simulink model "MOBATSim"  (R2020a)
settings: Solver=VariableStepAuto  StartTime=0.0  StopTime=20  FixedStep=0.01  RelTol=1e-3
undefined symbols (not defined in the file): default_spacing, FI_distance, FI_speed, max_ac, meters, min_ac, SafeDistance, Sim_Ts, simSpeed, time_gap, Ts, v_set, Vehicle1, Vehicle10, Vehicle2, Vehicle3, Vehicle4, Vehicle5, Vehicle6, Vehicle7, Vehicle8, Vehicle9, verr_gain, vx_gain, xerr_gain
libraries: simulink x32, mpcadaslib x1, robotalgslib x1
(part 3 of 4)

== system MOBATSim/Vehicle Model 9/Longitudinal Speed Control ==
  note: Here the measured speed and the actual speed are the same
      | but it is designed to include the effects of the measurement errors
  note: The vehicle calculates the speed difference between the actual speed and the reference speed, then generates the acceleration command accordingly.
  Speed Reference : Inport
  Inter Vehicular Distance : Inport  Port=2
  Lead Speed : Inport  Port=3
  Driving Mode : Inport  Port=4
  Dist2Stop : Inport  Port=5
  Acceleration Command : Subsystem
  Distance to Stop Controller : Subsystem
  Platoon Controller : Subsystem
  Reference speed according to the driving mode : Subsystem
  Signal Specification1 : SignalSpecification  Dimensions=1
  Sum13 : Sum  Inputs=|+-
  Vehicle Dynamic Model : Subsystem
  Actual Speed : Outport  VectorParamsAs1DForOutWhenUnconnected=off
  Measured Speed : Outport  Port=2  VectorParamsAs1DForOutWhenUnconnected=off
  wires:
  Platoon Controller/1(ref speed) -> Distance to Stop Controller/1(Speed Ref from Platoon), Reference speed according to the driving mode/3(In3)
  Lead Speed/1 -> Platoon Controller/2(Lead Speed)
  Driving Mode/1 -> Acceleration Command/1(Driving Mode), Reference speed according to the driving mode/1(In1)
  Signal Specification1/1 -> Actual Speed/1
  Sum13/1 -> Acceleration Command/2(Speed Error)
  Inter Vehicular Distance/1 -> Platoon Controller/1(Inter Vehicular Distance)
  Dist2Stop/1 -> Distance to Stop Controller/2(Distance to Stop)
  Speed Reference/1 -> Reference speed according to the driving mode/2(In2)
  Distance to Stop Controller/1(ref speed) -> Reference speed according to the driving mode/4(In4)
  Reference speed according to the driving mode/1(Out1) -> Sum13/1
  Vehicle Dynamic Model/1(Vehicle Speed) -> Signal Specification1/1, Acceleration Command/3(Actual Speed), Sum13/2, Platoon Controller/3(Vehicle Speed), Measured Speed/1
  Acceleration Command/1(Acceleration Command) -> Vehicle Dynamic Model/1(Acceleration Command)

== system MOBATSim/Vehicle Model 1/Longitudinal Speed Control/Acceleration Command ==
  Driving Mode : Inport
  Speed Error : Inport  Port=2
  Actual Speed : Inport  Port=3
  Emergency Brake : Constant  Value=MinDeceleration
  Gear Logic : Stateflow chart  TreatAsAtomicUnit=on
  Multiport Switch3 : MultiPortSwitch  Inputs=4
  Saturation Dynamic : simulink/Discontinuities/Saturation Dynamic  OutMin=[]  OutMax=[]  OutDataTypeStr=Inherit: Same as second input  OutDataType=fixdt(1, 16)  OutScaling=2^-10  DoSatur=off
  Acceleration Command : Outport  VectorParamsAs1DForOutWhenUnconnected=off
  wires:
  Driving Mode/1 -> Multiport Switch3/1
  Speed Error/1 -> Saturation Dynamic/2
  Emergency Brake/1 -> Saturation Dynamic/3, Multiport Switch3/4
  Saturation Dynamic/1 -> Multiport Switch3/5, Multiport Switch3/2, Multiport Switch3/3
  Actual Speed/1 -> Gear Logic/1(speed)
  Multiport Switch3/1 -> Acceleration Command/1
  Gear Logic/1(maxAcc) -> Saturation Dynamic/1

== system MOBATSim/Vehicle Model 1/Longitudinal Speed Control/Distance to Stop Controller ==
  Speed Ref from Platoon : Inport
  Distance to Stop : Inport  Port=2
  Gain : Gain  Gain=0.02
  Multiport Switch2 : MultiPortSwitch  DataPortOrder=Zero-based contiguous  Inputs=2  zeroidx=on
  Relational Operator : RelationalOperator  Operator=<=  OutDataTypeStr=boolean  RndMeth=Simplest
  ref speed : Outport  VectorParamsAs1DForOutWhenUnconnected=off
  wires:
  Distance to Stop/1 -> Gain/1
  Speed Ref from Platoon/1 -> Relational Operator/1, Multiport Switch2/3
  Gain/1 -> Relational Operator/2, Multiport Switch2/2
  Multiport Switch2/1 -> ref speed/1
  Relational Operator/1 -> Multiport Switch2/1

== system MOBATSim/Vehicle Model 1/Longitudinal Speed Control/Platoon Controller ==
  Inter Vehicular Distance : Inport
  Lead Speed : Inport  Port=2
  Vehicle Speed : Inport  Port=3
  Compare To Constant : simulink/Logic and Bit Operations/Compare To Constant  relop=>  const=2  OutDataTypeStr=uint8
  Constant : Constant  Value=meters
  Gain : Gain  Gain=1.4
  Multiport Switch : MultiPortSwitch  DataPortOrder=Zero-based contiguous  Inputs=2  zeroidx=on
  PID Controller5 : simulink/Continuous/PID Controller  Controller=PID  Form=Parallel  TimeDomain=Continuous-time  UseExternalTs=off  SampleTime=-1  IntegratorMethod=Forward Euler  FilterMethod=Forward Euler  ControllerParametersSource=internal  P=2.0341199375219  I=0.0356576460366845  D=2.08363010404189  UseFilter=on  N=233.214579742572  TunerSelectOption=Transfer Function Based (PID Tuner App)  InitialConditionSource=internal  InitialConditionForIntegrator=0  InitialConditionForFilter=0  DifferentiatorICPrevScaledInput=0  ExternalReset=none  TrackingMode=off  Kt=1  LimitOutput=on  UpperSaturationLimit=100  LowerSaturationLimit=-100  LinearizeAsGain=on  AntiWindupMode=clamping  Kb=1  POutMin=[]  POutMax=[]  IOutMin=[]  IOutMax=[]  DOutMin=[]  DOutMax=[]  NOutMin=[]  NOutMax=[]  SumOutMin=[]  SumOutMax=[]  SaturationOutMin=[]  SaturationOutMax=[]  PParamMin=[]  PParamMax=[]  IParamMin=[]  IParamMax=[]  DParamMin=[]  DParamMax=[]  NParamMin=[]  NParamMax=[]  KbParamMin=[]  KbParamMax=[]  KtParamMin=[]  KtParamMax=[]  KbOutMin=[]  KbOutMax=[]  KtOutMin=[]  KtOutMax=[]  IntegratorOutMin=[]  IntegratorOutMax=[]  FilterOutMin=[]  FilterOutMax=[]  SumI1OutMin=[]  SumI1OutMax=[]  SumI2OutMin=[]  SumI2OutMax=[]  SumI3OutMin=[]  SumI3OutMax=[]  SumI4OutMin=[]  SumI4OutMax=[]  SumDOutMin=[]  SumDOutMax=[]  DifferentiatorOutMin=[]  DifferentiatorOutMax=[]  FilterDiffOutCoefMin=[]  FilterDiffOutCoefMax=[]  ReciprocalOutMin=[]  ReciprocalOutMax=[]  SumDenOutMin=[]  SumDenOutMax=[]  SumNumOutMin=[]  SumNumOutMax=[]  DivideOutMin=[]  DivideOutMax=[]  UdiffTsProdOutMin=[]  UdiffTsProdOutMax=[]  NTsProdOutMin=[]  NTsProdOutMax=[]  UintegralTsProdOutMin=[]  UintegralTsProdOutMax=[]  UngainTsProdOutMin=[]  UngainTsProdOutMax=[]  IntegratorContinuousStateAttributes=''  IntegratorStateMustResolveToSignalObject=off  IntegratorRTWStateStorageClass=Auto  FilterContinuousStateAttributes=''  FilterStateMustResolveToSignalObject=off  FilterRTWStateStorageClass=Auto  ParallelPVariant=InternalParameters  IdealPVariant=Disabled  IVariant=InternalParameters  DVariant=InternalParameters  IntegratorVariant=Continuous  SatVariant=Enabled  AWVariant=ContClampingParallel  PCopyVariant=Disabled  TRVariant=Disabled  FdbkBlocksVariant=Forward  IdealPFdbkVariant=Disabled  SatFdbkVariant=Disabled  DerivativeFilterVariant=ContFilter  NVariant=InternalParameters  NCopyVariant=Disabled  FilterICVariant=InternalICsFilter  IntegratorICVariant=InternalICs  ExternalResetVariant=Disabled  TRSumVariant=Passthrough  SumFdbkVariant=Disabled  SumVariant=Sum_PID  TsampFilterVariant=InternalTs  TsampNgainVariant=Passthrough  TsampIntegralVariant=Passthrough
  Sum : Sum  Inputs=|-+
  Sum1 : Sum  Inputs=|++
  Sum2 : Sum  Inputs=|+-
  Transfer Fcn : TransferFcn  Numerator=[0.05]  Denominator=[1 2]
  ref speed : Outport  VectorParamsAs1DForOutWhenUnconnected=off
  wires:
  Transfer Fcn/1 -> PID Controller5/1
  Vehicle Speed/1 -> Gain/1, Sum/1
  PID Controller5/1 -> Multiport Switch/2
  Sum/1 -> Compare To Constant/1
  Multiport Switch/1 -> ref speed/1
  Compare To Constant/1 -> Multiport Switch/1
  Lead Speed/1 -> Sum/2, Multiport Switch/3
  Constant/1 -> Sum1/1
  Sum1/1 -> Sum2/2
  Gain/1 -> Sum1/2
  Sum2/1 -> Transfer Fcn/1
  Inter Vehicular Distance/1 -> Sum2/1

== system MOBATSim/Vehicle Model 1/Longitudinal Speed Control/Reference speed according to the driving mode ==
  In1 : Inport
  In2 : Inport  Port=2
  In3 : Inport  Port=3
  In4 : Inport  Port=4
  Constant1 : Constant  Value=0
  Max Speed : Saturate  UpperLimit=maxSpeed  LowerLimit=-100
  Multiport Switch : MultiPortSwitch  Inputs=4
  Out1 : Outport
  wires:
  Constant1/1 -> Multiport Switch/4
  Multiport Switch/1 -> Max Speed/1
  In1/1 -> Multiport Switch/1
  In3/1 -> Multiport Switch/3
  In2/1 -> Multiport Switch/2
  Max Speed/1 -> Out1/1
  In4/1 -> Multiport Switch/5

== system MOBATSim/Vehicle Model 1/Longitudinal Speed Control/Vehicle Dynamic Model ==
  Acceleration Command : Inport
  Integrator : Integrator  LimitOutput=on  LowerSaturationLimit=0
  Vehicle Acc to Speed Dynamics : TransferFcn  Denominator=[0.5 1]
  Vehicle Speed : Outport
  wires:
  Vehicle Acc to Speed Dynamics/1 -> Integrator/1
  Integrator/1 -> Vehicle Speed/1
  Acceleration Command/1 -> Vehicle Acc to Speed Dynamics/1

== system MOBATSim/Vehicle Model 10/Longitudinal Speed Control/Acceleration Command ==
  Driving Mode : Inport
  Speed Error : Inport  Port=2
  Actual Speed : Inport  Port=3
  Emergency Brake : Constant  Value=MinDeceleration
  Gear Logic : Stateflow chart  TreatAsAtomicUnit=on
  Multiport Switch3 : MultiPortSwitch  Inputs=4
  Saturation Dynamic : simulink/Discontinuities/Saturation Dynamic  OutMin=[]  OutMax=[]  OutDataTypeStr=Inherit: Same as second input  OutDataType=fixdt(1, 16)  OutScaling=2^-10  DoSatur=off
  Acceleration Command : Outport  VectorParamsAs1DForOutWhenUnconnected=off
  wires:
  Driving Mode/1 -> Multiport Switch3/1
  Speed Error/1 -> Saturation Dynamic/2
  Emergency Brake/1 -> Saturation Dynamic/3, Multiport Switch3/4
  Saturation Dynamic/1 -> Multiport Switch3/5, Multiport Switch3/2, Multiport Switch3/3
  Actual Speed/1 -> Gear Logic/1(speed)
  Multiport Switch3/1 -> Acceleration Command/1
  Gear Logic/1(maxAcc) -> Saturation Dynamic/1

== system MOBATSim/Vehicle Model 10/Longitudinal Speed Control/Distance to Stop Controller ==
  Speed Ref from Platoon : Inport
  Distance to Stop : Inport  Port=2
  Gain : Gain  Gain=0.02
  Multiport Switch2 : MultiPortSwitch  DataPortOrder=Zero-based contiguous  Inputs=2  zeroidx=on
  Relational Operator : RelationalOperator  Operator=<=  OutDataTypeStr=boolean  RndMeth=Simplest
  ref speed : Outport  VectorParamsAs1DForOutWhenUnconnected=off
  wires:
  Distance to Stop/1 -> Gain/1
  Speed Ref from Platoon/1 -> Relational Operator/1, Multiport Switch2/3
  Gain/1 -> Relational Operator/2, Multiport Switch2/2
  Multiport Switch2/1 -> ref speed/1
  Relational Operator/1 -> Multiport Switch2/1

== system MOBATSim/Vehicle Model 10/Longitudinal Speed Control/Platoon Controller ==
  Inter Vehicular Distance : Inport
  Lead Speed : Inport  Port=2
  Vehicle Speed : Inport  Port=3
  Compare To Constant : simulink/Logic and Bit Operations/Compare To Constant  relop=>  const=2  OutDataTypeStr=uint8
  Constant : Constant  Value=meters
  Gain : Gain  Gain=1.4
  Multiport Switch : MultiPortSwitch  DataPortOrder=Zero-based contiguous  Inputs=2  zeroidx=on
  PID Controller5 : simulink/Continuous/PID Controller  Controller=PID  Form=Parallel  TimeDomain=Continuous-time  UseExternalTs=off  SampleTime=-1  IntegratorMethod=Forward Euler  FilterMethod=Forward Euler  ControllerParametersSource=internal  P=2.0341199375219  I=0.0356576460366845  D=2.08363010404189  UseFilter=on  N=233.214579742572  TunerSelectOption=Transfer Function Based (PID Tuner App)  InitialConditionSource=internal  InitialConditionForIntegrator=0  InitialConditionForFilter=0  DifferentiatorICPrevScaledInput=0  ExternalReset=none  TrackingMode=off  Kt=1  LimitOutput=on  UpperSaturationLimit=100  LowerSaturationLimit=-100  LinearizeAsGain=on  AntiWindupMode=clamping  Kb=1  POutMin=[]  POutMax=[]  IOutMin=[]  IOutMax=[]  DOutMin=[]  DOutMax=[]  NOutMin=[]  NOutMax=[]  SumOutMin=[]  SumOutMax=[]  SaturationOutMin=[]  SaturationOutMax=[]  PParamMin=[]  PParamMax=[]  IParamMin=[]  IParamMax=[]  DParamMin=[]  DParamMax=[]  NParamMin=[]  NParamMax=[]  KbParamMin=[]  KbParamMax=[]  KtParamMin=[]  KtParamMax=[]  KbOutMin=[]  KbOutMax=[]  KtOutMin=[]  KtOutMax=[]  IntegratorOutMin=[]  IntegratorOutMax=[]  FilterOutMin=[]  FilterOutMax=[]  SumI1OutMin=[]  SumI1OutMax=[]  SumI2OutMin=[]  SumI2OutMax=[]  SumI3OutMin=[]  SumI3OutMax=[]  SumI4OutMin=[]  SumI4OutMax=[]  SumDOutMin=[]  SumDOutMax=[]  DifferentiatorOutMin=[]  DifferentiatorOutMax=[]  FilterDiffOutCoefMin=[]  FilterDiffOutCoefMax=[]  ReciprocalOutMin=[]  ReciprocalOutMax=[]  SumDenOutMin=[]  SumDenOutMax=[]  SumNumOutMin=[]  SumNumOutMax=[]  DivideOutMin=[]  DivideOutMax=[]  UdiffTsProdOutMin=[]  UdiffTsProdOutMax=[]  NTsProdOutMin=[]  NTsProdOutMax=[]  UintegralTsProdOutMin=[]  UintegralTsProdOutMax=[]  UngainTsProdOutMin=[]  UngainTsProdOutMax=[]  IntegratorContinuousStateAttributes=''  IntegratorStateMustResolveToSignalObject=off  IntegratorRTWStateStorageClass=Auto  FilterContinuousStateAttributes=''  FilterStateMustResolveToSignalObject=off  FilterRTWStateStorageClass=Auto  ParallelPVariant=InternalParameters  IdealPVariant=Disabled  IVariant=InternalParameters  DVariant=InternalParameters  IntegratorVariant=Continuous  SatVariant=Enabled  AWVariant=ContClampingParallel  PCopyVariant=Disabled  TRVariant=Disabled  FdbkBlocksVariant=Forward  IdealPFdbkVariant=Disabled  SatFdbkVariant=Disabled  DerivativeFilterVariant=ContFilter  NVariant=InternalParameters  NCopyVariant=Disabled  FilterICVariant=InternalICsFilter  IntegratorICVariant=InternalICs  ExternalResetVariant=Disabled  TRSumVariant=Passthrough  SumFdbkVariant=Disabled  SumVariant=Sum_PID  TsampFilterVariant=InternalTs  TsampNgainVariant=Passthrough  TsampIntegralVariant=Passthrough
  Sum : Sum  Inputs=|-+
  Sum1 : Sum  Inputs=|++
  Sum2 : Sum  Inputs=|+-
  Transfer Fcn : TransferFcn  Numerator=[0.05]  Denominator=[1 2]
  ref speed : Outport  VectorParamsAs1DForOutWhenUnconnected=off
  wires:
  Transfer Fcn/1 -> PID Controller5/1
  Vehicle Speed/1 -> Gain/1, Sum/1
  PID Controller5/1 -> Multiport Switch/2
  Sum/1 -> Compare To Constant/1
  Multiport Switch/1 -> ref speed/1
  Compare To Constant/1 -> Multiport Switch/1
  Lead Speed/1 -> Sum/2, Multiport Switch/3
  Constant/1 -> Sum1/1
  Sum1/1 -> Sum2/2
  Gain/1 -> Sum1/2
  Sum2/1 -> Transfer Fcn/1
  Inter Vehicular Distance/1 -> Sum2/1

== system MOBATSim/Vehicle Model 10/Longitudinal Speed Control/Reference speed according to the driving mode ==
  In1 : Inport
  In2 : Inport  Port=2
  In3 : Inport  Port=3
  In4 : Inport  Port=4
  Constant1 : Constant  Value=0
  Max Speed : Saturate  UpperLimit=maxSpeed  LowerLimit=-100
  Multiport Switch : MultiPortSwitch  Inputs=4
  Out1 : Outport
  wires:
  Constant1/1 -> Multiport Switch/4
  Multiport Switch/1 -> Max Speed/1
  In1/1 -> Multiport Switch/1
  In3/1 -> Multiport Switch/3
  In2/1 -> Multiport Switch/2
  Max Speed/1 -> Out1/1
  In4/1 -> Multiport Switch/5

== system MOBATSim/Vehicle Model 10/Longitudinal Speed Control/Vehicle Dynamic Model ==
  Acceleration Command : Inport
  Integrator : Integrator  LimitOutput=on  LowerSaturationLimit=0
  Vehicle Acc to Speed Dynamics : TransferFcn  Denominator=[0.5 1]
  Vehicle Speed : Outport
  wires:
  Vehicle Acc to Speed Dynamics/1 -> Integrator/1
  Integrator/1 -> Vehicle Speed/1
  Acceleration Command/1 -> Vehicle Acc to Speed Dynamics/1

== system MOBATSim/Vehicle Model 2/Longitudinal Speed Control/Acceleration Command ==
  Driving Mode : Inport
  Speed Error : Inport  Port=2
  Actual Speed : Inport  Port=3
  Emergency Brake : Constant  Value=MinDeceleration
  Gear Logic : Stateflow chart  TreatAsAtomicUnit=on
  Multiport Switch3 : MultiPortSwitch  Inputs=4
  Saturation Dynamic : simulink/Discontinuities/Saturation Dynamic  OutMin=[]  OutMax=[]  OutDataTypeStr=Inherit: Same as second input  OutDataType=fixdt(1, 16)  OutScaling=2^-10  DoSatur=off
  Acceleration Command : Outport  VectorParamsAs1DForOutWhenUnconnected=off
  wires:
  Driving Mode/1 -> Multiport Switch3/1
  Speed Error/1 -> Saturation Dynamic/2
  Emergency Brake/1 -> Saturation Dynamic/3, Multiport Switch3/4
  Saturation Dynamic/1 -> Multiport Switch3/5, Multiport Switch3/2, Multiport Switch3/3
  Actual Speed/1 -> Gear Logic/1(speed)
  Multiport Switch3/1 -> Acceleration Command/1
  Gear Logic/1(maxAcc) -> Saturation Dynamic/1

== system MOBATSim/Vehicle Model 2/Longitudinal Speed Control/Distance to Stop Controller ==
  Speed Ref from Platoon : Inport
  Distance to Stop : Inport  Port=2
  Gain : Gain  Gain=0.02
  Multiport Switch2 : MultiPortSwitch  DataPortOrder=Zero-based contiguous  Inputs=2  zeroidx=on
  Relational Operator : RelationalOperator  Operator=<=  OutDataTypeStr=boolean  RndMeth=Simplest
  ref speed : Outport  VectorParamsAs1DForOutWhenUnconnected=off
  wires:
  Distance to Stop/1 -> Gain/1
  Speed Ref from Platoon/1 -> Relational Operator/1, Multiport Switch2/3
  Gain/1 -> Relational Operator/2, Multiport Switch2/2
  Multiport Switch2/1 -> ref speed/1
  Relational Operator/1 -> Multiport Switch2/1

== system MOBATSim/Vehicle Model 2/Longitudinal Speed Control/Platoon Controller ==
  Inter Vehicular Distance : Inport
  Lead Speed : Inport  Port=2
  Vehicle Speed : Inport  Port=3
  Compare To Constant : simulink/Logic and Bit Operations/Compare To Constant  relop=>  const=2  OutDataTypeStr=uint8
  Constant : Constant  Value=meters
  Gain : Gain  Gain=1.4
  Multiport Switch : MultiPortSwitch  DataPortOrder=Zero-based contiguous  Inputs=2  zeroidx=on
  PID Controller5 : simulink/Continuous/PID Controller  Controller=PID  Form=Parallel  TimeDomain=Continuous-time  UseExternalTs=off  SampleTime=-1  IntegratorMethod=Forward Euler  FilterMethod=Forward Euler  ControllerParametersSource=internal  P=2.0341199375219  I=0.0356576460366845  D=2.08363010404189  UseFilter=on  N=233.214579742572  TunerSelectOption=Transfer Function Based (PID Tuner App)  InitialConditionSource=internal  InitialConditionForIntegrator=0  InitialConditionForFilter=0  DifferentiatorICPrevScaledInput=0  ExternalReset=none  TrackingMode=off  Kt=1  LimitOutput=on  UpperSaturationLimit=100  LowerSaturationLimit=-100  LinearizeAsGain=on  AntiWindupMode=clamping  Kb=1  POutMin=[]  POutMax=[]  IOutMin=[]  IOutMax=[]  DOutMin=[]  DOutMax=[]  NOutMin=[]  NOutMax=[]  SumOutMin=[]  SumOutMax=[]  SaturationOutMin=[]  SaturationOutMax=[]  PParamMin=[]  PParamMax=[]  IParamMin=[]  IParamMax=[]  DParamMin=[]  DParamMax=[]  NParamMin=[]  NParamMax=[]  KbParamMin=[]  KbParamMax=[]  KtParamMin=[]  KtParamMax=[]  KbOutMin=[]  KbOutMax=[]  KtOutMin=[]  KtOutMax=[]  IntegratorOutMin=[]  IntegratorOutMax=[]  FilterOutMin=[]  FilterOutMax=[]  SumI1OutMin=[]  SumI1OutMax=[]  SumI2OutMin=[]  SumI2OutMax=[]  SumI3OutMin=[]  SumI3OutMax=[]  SumI4OutMin=[]  SumI4OutMax=[]  SumDOutMin=[]  SumDOutMax=[]  DifferentiatorOutMin=[]  DifferentiatorOutMax=[]  FilterDiffOutCoefMin=[]  FilterDiffOutCoefMax=[]  ReciprocalOutMin=[]  ReciprocalOutMax=[]  SumDenOutMin=[]  SumDenOutMax=[]  SumNumOutMin=[]  SumNumOutMax=[]  DivideOutMin=[]  DivideOutMax=[]  UdiffTsProdOutMin=[]  UdiffTsProdOutMax=[]  NTsProdOutMin=[]  NTsProdOutMax=[]  UintegralTsProdOutMin=[]  UintegralTsProdOutMax=[]  UngainTsProdOutMin=[]  UngainTsProdOutMax=[]  IntegratorContinuousStateAttributes=''  IntegratorStateMustResolveToSignalObject=off  IntegratorRTWStateStorageClass=Auto  FilterContinuousStateAttributes=''  FilterStateMustResolveToSignalObject=off  FilterRTWStateStorageClass=Auto  ParallelPVariant=InternalParameters  IdealPVariant=Disabled  IVariant=InternalParameters  DVariant=InternalParameters  IntegratorVariant=Continuous  SatVariant=Enabled  AWVariant=ContClampingParallel  PCopyVariant=Disabled  TRVariant=Disabled  FdbkBlocksVariant=Forward  IdealPFdbkVariant=Disabled  SatFdbkVariant=Disabled  DerivativeFilterVariant=ContFilter  NVariant=InternalParameters  NCopyVariant=Disabled  FilterICVariant=InternalICsFilter  IntegratorICVariant=InternalICs  ExternalResetVariant=Disabled  TRSumVariant=Passthrough  SumFdbkVariant=Disabled  SumVariant=Sum_PID  TsampFilterVariant=InternalTs  TsampNgainVariant=Passthrough  TsampIntegralVariant=Passthrough
  Sum : Sum  Inputs=|-+
  Sum1 : Sum  Inputs=|++
  Sum2 : Sum  Inputs=|+-
  Transfer Fcn : TransferFcn  Numerator=[0.05]  Denominator=[1 2]
  ref speed : Outport  VectorParamsAs1DForOutWhenUnconnected=off
  wires:
  Transfer Fcn/1 -> PID Controller5/1
  Vehicle Speed/1 -> Gain/1, Sum/1
  PID Controller5/1 -> Multiport Switch/2
  Sum/1 -> Compare To Constant/1
  Multiport Switch/1 -> ref speed/1
  Compare To Constant/1 -> Multiport Switch/1
  Lead Speed/1 -> Sum/2, Multiport Switch/3
  Constant/1 -> Sum1/1
  Sum1/1 -> Sum2/2
  Gain/1 -> Sum1/2
  Sum2/1 -> Transfer Fcn/1
  Inter Vehicular Distance/1 -> Sum2/1

== system MOBATSim/Vehicle Model 2/Longitudinal Speed Control/Reference speed according to the driving mode ==
  In1 : Inport
  In2 : Inport  Port=2
  In3 : Inport  Port=3
  In4 : Inport  Port=4
  Constant1 : Constant  Value=0
  Max Speed : Saturate  UpperLimit=maxSpeed  LowerLimit=-100
  Multiport Switch : MultiPortSwitch  Inputs=4
  Out1 : Outport
  wires:
  Constant1/1 -> Multiport Switch/4
  Multiport Switch/1 -> Max Speed/1
  In1/1 -> Multiport Switch/1
  In3/1 -> Multiport Switch/3
  In2/1 -> Multiport Switch/2
  Max Speed/1 -> Out1/1
  In4/1 -> Multiport Switch/5

== system MOBATSim/Vehicle Model 2/Longitudinal Speed Control/Vehicle Dynamic Model ==
  Acceleration Command : Inport
  Integrator : Integrator  LimitOutput=on  LowerSaturationLimit=0
  Vehicle Acc to Speed Dynamics : TransferFcn  Denominator=[0.5 1]
  Vehicle Speed : Outport
  wires:
  Vehicle Acc to Speed Dynamics/1 -> Integrator/1
  Integrator/1 -> Vehicle Speed/1
  Acceleration Command/1 -> Vehicle Acc to Speed Dynamics/1

== system MOBATSim/Vehicle Model 3/Longitudinal Speed Control/Acceleration Command ==
  Driving Mode : Inport
  Speed Error : Inport  Port=2
  Actual Speed : Inport  Port=3
  Emergency Brake : Constant  Value=MinDeceleration
  Gear Logic : Stateflow chart  TreatAsAtomicUnit=on
  Multiport Switch3 : MultiPortSwitch  Inputs=4
  Saturation Dynamic : simulink/Discontinuities/Saturation Dynamic  OutMin=[]  OutMax=[]  OutDataTypeStr=Inherit: Same as second input  OutDataType=fixdt(1, 16)  OutScaling=2^-10  DoSatur=off
  Acceleration Command : Outport  VectorParamsAs1DForOutWhenUnconnected=off
  wires:
  Driving Mode/1 -> Multiport Switch3/1
  Speed Error/1 -> Saturation Dynamic/2
  Emergency Brake/1 -> Saturation Dynamic/3, Multiport Switch3/4
  Saturation Dynamic/1 -> Multiport Switch3/5, Multiport Switch3/2, Multiport Switch3/3
  Actual Speed/1 -> Gear Logic/1(speed)
  Multiport Switch3/1 -> Acceleration Command/1
  Gear Logic/1(maxAcc) -> Saturation Dynamic/1

== system MOBATSim/Vehicle Model 3/Longitudinal Speed Control/Distance to Stop Controller ==
  Speed Ref from Platoon : Inport
  Distance to Stop : Inport  Port=2
  Gain : Gain  Gain=0.02
  Multiport Switch2 : MultiPortSwitch  DataPortOrder=Zero-based contiguous  Inputs=2  zeroidx=on
  Relational Operator : RelationalOperator  Operator=<=  OutDataTypeStr=boolean  RndMeth=Simplest
  ref speed : Outport  VectorParamsAs1DForOutWhenUnconnected=off
  wires:
  Distance to Stop/1 -> Gain/1
  Speed Ref from Platoon/1 -> Relational Operator/1, Multiport Switch2/3
  Gain/1 -> Relational Operator/2, Multiport Switch2/2
  Multiport Switch2/1 -> ref speed/1
  Relational Operator/1 -> Multiport Switch2/1

== system MOBATSim/Vehicle Model 3/Longitudinal Speed Control/Platoon Controller ==
  Inter Vehicular Distance : Inport
  Lead Speed : Inport  Port=2
  Vehicle Speed : Inport  Port=3
  Compare To Constant : simulink/Logic and Bit Operations/Compare To Constant  relop=>  const=2  OutDataTypeStr=uint8
  Constant : Constant  Value=meters
  Gain : Gain  Gain=1.4
  Multiport Switch : MultiPortSwitch  DataPortOrder=Zero-based contiguous  Inputs=2  zeroidx=on
  PID Controller5 : simulink/Continuous/PID Controller  Controller=PID  Form=Parallel  TimeDomain=Continuous-time  UseExternalTs=off  SampleTime=-1  IntegratorMethod=Forward Euler  FilterMethod=Forward Euler  ControllerParametersSource=internal  P=2.0341199375219  I=0.0356576460366845  D=2.08363010404189  UseFilter=on  N=233.214579742572  TunerSelectOption=Transfer Function Based (PID Tuner App)  InitialConditionSource=internal  InitialConditionForIntegrator=0  InitialConditionForFilter=0  DifferentiatorICPrevScaledInput=0  ExternalReset=none  TrackingMode=off  Kt=1  LimitOutput=on  UpperSaturationLimit=100  LowerSaturationLimit=-100  LinearizeAsGain=on  AntiWindupMode=clamping  Kb=1  POutMin=[]  POutMax=[]  IOutMin=[]  IOutMax=[]  DOutMin=[]  DOutMax=[]  NOutMin=[]  NOutMax=[]  SumOutMin=[]  SumOutMax=[]  SaturationOutMin=[]  SaturationOutMax=[]  PParamMin=[]  PParamMax=[]  IParamMin=[]  IParamMax=[]  DParamMin=[]  DParamMax=[]  NParamMin=[]  NParamMax=[]  KbParamMin=[]  KbParamMax=[]  KtParamMin=[]  KtParamMax=[]  KbOutMin=[]  KbOutMax=[]  KtOutMin=[]  KtOutMax=[]  IntegratorOutMin=[]  IntegratorOutMax=[]  FilterOutMin=[]  FilterOutMax=[]  SumI1OutMin=[]  SumI1OutMax=[]  SumI2OutMin=[]  SumI2OutMax=[]  SumI3OutMin=[]  SumI3OutMax=[]  SumI4OutMin=[]  SumI4OutMax=[]  SumDOutMin=[]  SumDOutMax=[]  DifferentiatorOutMin=[]  DifferentiatorOutMax=[]  FilterDiffOutCoefMin=[]  FilterDiffOutCoefMax=[]  ReciprocalOutMin=[]  ReciprocalOutMax=[]  SumDenOutMin=[]  SumDenOutMax=[]  SumNumOutMin=[]  SumNumOutMax=[]  DivideOutMin=[]  DivideOutMax=[]  UdiffTsProdOutMin=[]  UdiffTsProdOutMax=[]  NTsProdOutMin=[]  NTsProdOutMax=[]  UintegralTsProdOutMin=[]  UintegralTsProdOutMax=[]  UngainTsProdOutMin=[]  UngainTsProdOutMax=[]  IntegratorContinuousStateAttributes=''  IntegratorStateMustResolveToSignalObject=off  IntegratorRTWStateStorageClass=Auto  FilterContinuousStateAttributes=''  FilterStateMustResolveToSignalObject=off  FilterRTWStateStorageClass=Auto  ParallelPVariant=InternalParameters  IdealPVariant=Disabled  IVariant=InternalParameters  DVariant=InternalParameters  IntegratorVariant=Continuous  SatVariant=Enabled  AWVariant=ContClampingParallel  PCopyVariant=Disabled  TRVariant=Disabled  FdbkBlocksVariant=Forward  IdealPFdbkVariant=Disabled  SatFdbkVariant=Disabled  DerivativeFilterVariant=ContFilter  NVariant=InternalParameters  NCopyVariant=Disabled  FilterICVariant=InternalICsFilter  IntegratorICVariant=InternalICs  ExternalResetVariant=Disabled  TRSumVariant=Passthrough  SumFdbkVariant=Disabled  SumVariant=Sum_PID  TsampFilterVariant=InternalTs  TsampNgainVariant=Passthrough  TsampIntegralVariant=Passthrough
  Sum : Sum  Inputs=|-+
  Sum1 : Sum  Inputs=|++
  Sum2 : Sum  Inputs=|+-
  Transfer Fcn : TransferFcn  Numerator=[0.05]  Denominator=[1 2]
  ref speed : Outport  VectorParamsAs1DForOutWhenUnconnected=off
  wires:
  Transfer Fcn/1 -> PID Controller5/1
  Vehicle Speed/1 -> Gain/1, Sum/1
  PID Controller5/1 -> Multiport Switch/2
  Sum/1 -> Compare To Constant/1
  Multiport Switch/1 -> ref speed/1
  Compare To Constant/1 -> Multiport Switch/1
  Lead Speed/1 -> Sum/2, Multiport Switch/3
  Constant/1 -> Sum1/1
  Sum1/1 -> Sum2/2
  Gain/1 -> Sum1/2
  Sum2/1 -> Transfer Fcn/1
  Inter Vehicular Distance/1 -> Sum2/1

== system MOBATSim/Vehicle Model 3/Longitudinal Speed Control/Reference speed according to the driving mode ==
  In1 : Inport
  In2 : Inport  Port=2
  In3 : Inport  Port=3
  In4 : Inport  Port=4
  Constant1 : Constant  Value=0
  Max Speed : Saturate  UpperLimit=maxSpeed  LowerLimit=-100
  Multiport Switch : MultiPortSwitch  Inputs=4
  Out1 : Outport
  wires:
  Constant1/1 -> Multiport Switch/4
  Multiport Switch/1 -> Max Speed/1
  In1/1 -> Multiport Switch/1
  In3/1 -> Multiport Switch/3
  In2/1 -> Multiport Switch/2
  Max Speed/1 -> Out1/1
  In4/1 -> Multiport Switch/5

== system MOBATSim/Vehicle Model 3/Longitudinal Speed Control/Vehicle Dynamic Model ==
  Acceleration Command : Inport
  Integrator : Integrator  LimitOutput=on  LowerSaturationLimit=0
  Vehicle Acc to Speed Dynamics : TransferFcn  Denominator=[0.5 1]
  Vehicle Speed : Outport
  wires:
  Vehicle Acc to Speed Dynamics/1 -> Integrator/1
  Integrator/1 -> Vehicle Speed/1
  Acceleration Command/1 -> Vehicle Acc to Speed Dynamics/1

== system MOBATSim/Vehicle Model 4/Longitudinal Speed Control/Acceleration Command ==
  Driving Mode : Inport
  Speed Error : Inport  Port=2
  Actual Speed : Inport  Port=3
  Emergency Brake : Constant  Value=MinDeceleration
  Gear Logic : Stateflow chart  TreatAsAtomicUnit=on
  Multiport Switch3 : MultiPortSwitch  Inputs=4
  Saturation Dynamic : simulink/Discontinuities/Saturation Dynamic  OutMin=[]  OutMax=[]  OutDataTypeStr=Inherit: Same as second input  OutDataType=fixdt(1, 16)  OutScaling=2^-10  DoSatur=off
  Acceleration Command : Outport  VectorParamsAs1DForOutWhenUnconnected=off
  wires:
  Driving Mode/1 -> Multiport Switch3/1
  Speed Error/1 -> Saturation Dynamic/2
  Emergency Brake/1 -> Saturation Dynamic/3, Multiport Switch3/4
  Saturation Dynamic/1 -> Multiport Switch3/5, Multiport Switch3/2, Multiport Switch3/3
  Actual Speed/1 -> Gear Logic/1(speed)
  Multiport Switch3/1 -> Acceleration Command/1
  Gear Logic/1(maxAcc) -> Saturation Dynamic/1

== system MOBATSim/Vehicle Model 4/Longitudinal Speed Control/Distance to Stop Controller ==
  Speed Ref from Platoon : Inport
  Distance to Stop : Inport  Port=2
  Gain : Gain  Gain=0.02
  Multiport Switch2 : MultiPortSwitch  DataPortOrder=Zero-based contiguous  Inputs=2  zeroidx=on
  Relational Operator : RelationalOperator  Operator=<=  OutDataTypeStr=boolean  RndMeth=Simplest
  ref speed : Outport  VectorParamsAs1DForOutWhenUnconnected=off
  wires:
  Distance to Stop/1 -> Gain/1
  Speed Ref from Platoon/1 -> Relational Operator/1, Multiport Switch2/3
  Gain/1 -> Relational Operator/2, Multiport Switch2/2
  Multiport Switch2/1 -> ref speed/1
  Relational Operator/1 -> Multiport Switch2/1

== system MOBATSim/Vehicle Model 4/Longitudinal Speed Control/Platoon Controller ==
  Inter Vehicular Distance : Inport
  Lead Speed : Inport  Port=2
  Vehicle Speed : Inport  Port=3
  Compare To Constant : simulink/Logic and Bit Operations/Compare To Constant  relop=>  const=2  OutDataTypeStr=uint8
  Constant : Constant  Value=meters
  Gain : Gain  Gain=1.4
  Multiport Switch : MultiPortSwitch  DataPortOrder=Zero-based contiguous  Inputs=2  zeroidx=on
  PID Controller5 : simulink/Continuous/PID Controller  Controller=PID  Form=Parallel  TimeDomain=Continuous-time  UseExternalTs=off  SampleTime=-1  IntegratorMethod=Forward Euler  FilterMethod=Forward Euler  ControllerParametersSource=internal  P=2.0341199375219  I=0.0356576460366845  D=2.08363010404189  UseFilter=on  N=233.214579742572  TunerSelectOption=Transfer Function Based (PID Tuner App)  InitialConditionSource=internal  InitialConditionForIntegrator=0  InitialConditionForFilter=0  DifferentiatorICPrevScaledInput=0  ExternalReset=none  TrackingMode=off  Kt=1  LimitOutput=on  UpperSaturationLimit=100  LowerSaturationLimit=-100  LinearizeAsGain=on  AntiWindupMode=clamping  Kb=1  POutMin=[]  POutMax=[]  IOutMin=[]  IOutMax=[]  DOutMin=[]  DOutMax=[]  NOutMin=[]  NOutMax=[]  SumOutMin=[]  SumOutMax=[]  SaturationOutMin=[]  SaturationOutMax=[]  PParamMin=[]  PParamMax=[]  IParamMin=[]  IParamMax=[]  DParamMin=[]  DParamMax=[]  NParamMin=[]  NParamMax=[]  KbParamMin=[]  KbParamMax=[]  KtParamMin=[]  KtParamMax=[]  KbOutMin=[]  KbOutMax=[]  KtOutMin=[]  KtOutMax=[]  IntegratorOutMin=[]  IntegratorOutMax=[]  FilterOutMin=[]  FilterOutMax=[]  SumI1OutMin=[]  SumI1OutMax=[]  SumI2OutMin=[]  SumI2OutMax=[]  SumI3OutMin=[]  SumI3OutMax=[]  SumI4OutMin=[]  SumI4OutMax=[]  SumDOutMin=[]  SumDOutMax=[]  DifferentiatorOutMin=[]  DifferentiatorOutMax=[]  FilterDiffOutCoefMin=[]  FilterDiffOutCoefMax=[]  ReciprocalOutMin=[]  ReciprocalOutMax=[]  SumDenOutMin=[]  SumDenOutMax=[]  SumNumOutMin=[]  SumNumOutMax=[]  DivideOutMin=[]  DivideOutMax=[]  UdiffTsProdOutMin=[]  UdiffTsProdOutMax=[]  NTsProdOutMin=[]  NTsProdOutMax=[]  UintegralTsProdOutMin=[]  UintegralTsProdOutMax=[]  UngainTsProdOutMin=[]  UngainTsProdOutMax=[]  IntegratorContinuousStateAttributes=''  IntegratorStateMustResolveToSignalObject=off  IntegratorRTWStateStorageClass=Auto  FilterContinuousStateAttributes=''  FilterStateMustResolveToSignalObject=off  FilterRTWStateStorageClass=Auto  ParallelPVariant=InternalParameters  IdealPVariant=Disabled  IVariant=InternalParameters  DVariant=InternalParameters  IntegratorVariant=Continuous  SatVariant=Enabled  AWVariant=ContClampingParallel  PCopyVariant=Disabled  TRVariant=Disabled  FdbkBlocksVariant=Forward  IdealPFdbkVariant=Disabled  SatFdbkVariant=Disabled  DerivativeFilterVariant=ContFilter  NVariant=InternalParameters  NCopyVariant=Disabled  FilterICVariant=InternalICsFilter  IntegratorICVariant=InternalICs  ExternalResetVariant=Disabled  TRSumVariant=Passthrough  SumFdbkVariant=Disabled  SumVariant=Sum_PID  TsampFilterVariant=InternalTs  TsampNgainVariant=Passthrough  TsampIntegralVariant=Passthrough
  Sum : Sum  Inputs=|-+
  Sum1 : Sum  Inputs=|++
  Sum2 : Sum  Inputs=|+-
  Transfer Fcn : TransferFcn  Numerator=[0.05]  Denominator=[1 2]
  ref speed : Outport  VectorParamsAs1DForOutWhenUnconnected=off
  wires:
  Transfer Fcn/1 -> PID Controller5/1
  Vehicle Speed/1 -> Gain/1, Sum/1
  PID Controller5/1 -> Multiport Switch/2
  Sum/1 -> Compare To Constant/1
  Multiport Switch/1 -> ref speed/1
  Compare To Constant/1 -> Multiport Switch/1
  Lead Speed/1 -> Sum/2, Multiport Switch/3
  Constant/1 -> Sum1/1
  Sum1/1 -> Sum2/2
  Gain/1 -> Sum1/2
  Sum2/1 -> Transfer Fcn/1
  Inter Vehicular Distance/1 -> Sum2/1

== system MOBATSim/Vehicle Model 4/Longitudinal Speed Control/Reference speed according to the driving mode ==
  In1 : Inport
  In2 : Inport  Port=2
  In3 : Inport  Port=3
  In4 : Inport  Port=4
  Constant1 : Constant  Value=0
  Max Speed : Saturate  UpperLimit=maxSpeed  LowerLimit=-100
  Multiport Switch : MultiPortSwitch  Inputs=4
  Out1 : Outport
  wires:
  Constant1/1 -> Multiport Switch/4
  Multiport Switch/1 -> Max Speed/1
  In1/1 -> Multiport Switch/1
  In3/1 -> Multiport Switch/3
  In2/1 -> Multiport Switch/2
  Max Speed/1 -> Out1/1
  In4/1 -> Multiport Switch/5

== system MOBATSim/Vehicle Model 4/Longitudinal Speed Control/Vehicle Dynamic Model ==
  Acceleration Command : Inport
  Integrator : Integrator  LimitOutput=on  LowerSaturationLimit=0
  Vehicle Acc to Speed Dynamics : TransferFcn  Denominator=[0.5 1]
  Vehicle Speed : Outport
  wires:
  Vehicle Acc to Speed Dynamics/1 -> Integrator/1
  Integrator/1 -> Vehicle Speed/1
  Acceleration Command/1 -> Vehicle Acc to Speed Dynamics/1

== system MOBATSim/Vehicle Model 5/Longitudinal Speed Control/Acceleration Command ==
  Driving Mode : Inport
  Speed Error : Inport  Port=2
  Actual Speed : Inport  Port=3
  Emergency Brake : Constant  Value=MinDeceleration
  Gear Logic : Stateflow chart  TreatAsAtomicUnit=on
  Multiport Switch3 : MultiPortSwitch  Inputs=4
  Saturation Dynamic : simulink/Discontinuities/Saturation Dynamic  OutMin=[]  OutMax=[]  OutDataTypeStr=Inherit: Same as second input  OutDataType=fixdt(1, 16)  OutScaling=2^-10  DoSatur=off
  Acceleration Command : Outport  VectorParamsAs1DForOutWhenUnconnected=off
  wires:
  Driving Mode/1 -> Multiport Switch3/1
  Speed Error/1 -> Saturation Dynamic/2
  Emergency Brake/1 -> Saturation Dynamic/3, Multiport Switch3/4
  Saturation Dynamic/1 -> Multiport Switch3/5, Multiport Switch3/2, Multiport Switch3/3
  Actual Speed/1 -> Gear Logic/1(speed)
  Multiport Switch3/1 -> Acceleration Command/1
  Gear Logic/1(maxAcc) -> Saturation Dynamic/1

== system MOBATSim/Vehicle Model 5/Longitudinal Speed Control/Distance to Stop Controller ==
  Speed Ref from Platoon : Inport
  Distance to Stop : Inport  Port=2
  Gain : Gain  Gain=0.02
  Multiport Switch2 : MultiPortSwitch  DataPortOrder=Zero-based contiguous  Inputs=2  zeroidx=on
  Relational Operator : RelationalOperator  Operator=<=  OutDataTypeStr=boolean  RndMeth=Simplest
  ref speed : Outport  VectorParamsAs1DForOutWhenUnconnected=off
  wires:
  Distance to Stop/1 -> Gain/1
  Speed Ref from Platoon/1 -> Relational Operator/1, Multiport Switch2/3
  Gain/1 -> Relational Operator/2, Multiport Switch2/2
  Multiport Switch2/1 -> ref speed/1
  Relational Operator/1 -> Multiport Switch2/1

== system MOBATSim/Vehicle Model 5/Longitudinal Speed Control/Platoon Controller ==
  Inter Vehicular Distance : Inport
  Lead Speed : Inport  Port=2
  Vehicle Speed : Inport  Port=3
  Compare To Constant : simulink/Logic and Bit Operations/Compare To Constant  relop=>  const=2  OutDataTypeStr=uint8
  Constant : Constant  Value=meters
  Gain : Gain  Gain=1.4
  Multiport Switch : MultiPortSwitch  DataPortOrder=Zero-based contiguous  Inputs=2  zeroidx=on
  PID Controller5 : simulink/Continuous/PID Controller  Controller=PID  Form=Parallel  TimeDomain=Continuous-time  UseExternalTs=off  SampleTime=-1  IntegratorMethod=Forward Euler  FilterMethod=Forward Euler  ControllerParametersSource=internal  P=2.0341199375219  I=0.0356576460366845  D=2.08363010404189  UseFilter=on  N=233.214579742572  TunerSelectOption=Transfer Function Based (PID Tuner App)  InitialConditionSource=internal  InitialConditionForIntegrator=0  InitialConditionForFilter=0  DifferentiatorICPrevScaledInput=0  ExternalReset=none  TrackingMode=off  Kt=1  LimitOutput=on  UpperSaturationLimit=100  LowerSaturationLimit=-100  LinearizeAsGain=on  AntiWindupMode=clamping  Kb=1  POutMin=[]  POutMax=[]  IOutMin=[]  IOutMax=[]  DOutMin=[]  DOutMax=[]  NOutMin=[]  NOutMax=[]  SumOutMin=[]  SumOutMax=[]  SaturationOutMin=[]  SaturationOutMax=[]  PParamMin=[]  PParamMax=[]  IParamMin=[]  IParamMax=[]  DParamMin=[]  DParamMax=[]  NParamMin=[]  NParamMax=[]  KbParamMin=[]  KbParamMax=[]  KtParamMin=[]  KtParamMax=[]  KbOutMin=[]  KbOutMax=[]  KtOutMin=[]  KtOutMax=[]  IntegratorOutMin=[]  IntegratorOutMax=[]  FilterOutMin=[]  FilterOutMax=[]  SumI1OutMin=[]  SumI1OutMax=[]  SumI2OutMin=[]  SumI2OutMax=[]  SumI3OutMin=[]  SumI3OutMax=[]  SumI4OutMin=[]  SumI4OutMax=[]  SumDOutMin=[]  SumDOutMax=[]  DifferentiatorOutMin=[]  DifferentiatorOutMax=[]  FilterDiffOutCoefMin=[]  FilterDiffOutCoefMax=[]  ReciprocalOutMin=[]  ReciprocalOutMax=[]  SumDenOutMin=[]  SumDenOutMax=[]  SumNumOutMin=[]  SumNumOutMax=[]  DivideOutMin=[]  DivideOutMax=[]  UdiffTsProdOutMin=[]  UdiffTsProdOutMax=[]  NTsProdOutMin=[]  NTsProdOutMax=[]  UintegralTsProdOutMin=[]  UintegralTsProdOutMax=[]  UngainTsProdOutMin=[]  UngainTsProdOutMax=[]  IntegratorContinuousStateAttributes=''  IntegratorStateMustResolveToSignalObject=off  IntegratorRTWStateStorageClass=Auto  FilterContinuousStateAttributes=''  FilterStateMustResolveToSignalObject=off  FilterRTWStateStorageClass=Auto  ParallelPVariant=InternalParameters  IdealPVariant=Disabled  IVariant=InternalParameters  DVariant=InternalParameters  IntegratorVariant=Continuous  SatVariant=Enabled  AWVariant=ContClampingParallel  PCopyVariant=Disabled  TRVariant=Disabled  FdbkBlocksVariant=Forward  IdealPFdbkVariant=Disabled  SatFdbkVariant=Disabled  DerivativeFilterVariant=ContFilter  NVariant=InternalParameters  NCopyVariant=Disabled  FilterICVariant=InternalICsFilter  IntegratorICVariant=InternalICs  ExternalResetVariant=Disabled  TRSumVariant=Passthrough  SumFdbkVariant=Disabled  SumVariant=Sum_PID  TsampFilterVariant=InternalTs  TsampNgainVariant=Passthrough  TsampIntegralVariant=Passthrough
  Sum : Sum  Inputs=|-+
  Sum1 : Sum  Inputs=|++
  Sum2 : Sum  Inputs=|+-
  Transfer Fcn : TransferFcn  Numerator=[0.05]  Denominator=[1 2]
  ref speed : Outport  VectorParamsAs1DForOutWhenUnconnected=off
  wires:
  Transfer Fcn/1 -> PID Controller5/1
  Vehicle Speed/1 -> Gain/1, Sum/1
  PID Controller5/1 -> Multiport Switch/2
  Sum/1 -> Compare To Constant/1
  Multiport Switch/1 -> ref speed/1
  Compare To Constant/1 -> Multiport Switch/1
  Lead Speed/1 -> Sum/2, Multiport Switch/3
  Constant/1 -> Sum1/1
  Sum1/1 -> Sum2/2
  Gain/1 -> Sum1/2
  Sum2/1 -> Transfer Fcn/1
  Inter Vehicular Distance/1 -> Sum2/1

== system MOBATSim/Vehicle Model 5/Longitudinal Speed Control/Reference speed according to the driving mode ==
  In1 : Inport
  In2 : Inport  Port=2
  In3 : Inport  Port=3
  In4 : Inport  Port=4
  Constant1 : Constant  Value=0
  Max Speed : Saturate  UpperLimit=maxSpeed  LowerLimit=-100
  Multiport Switch : MultiPortSwitch  Inputs=4
  Out1 : Outport
  wires:
  Constant1/1 -> Multiport Switch/4
  Multiport Switch/1 -> Max Speed/1
  In1/1 -> Multiport Switch/1
  In3/1 -> Multiport Switch/3
  In2/1 -> Multiport Switch/2
  Max Speed/1 -> Out1/1
  In4/1 -> Multiport Switch/5

== system MOBATSim/Vehicle Model 5/Longitudinal Speed Control/Vehicle Dynamic Model ==
  Acceleration Command : Inport
  Integrator : Integrator  LimitOutput=on  LowerSaturationLimit=0
  Vehicle Acc to Speed Dynamics : TransferFcn  Denominator=[0.5 1]
  Vehicle Speed : Outport
  wires:
  Vehicle Acc to Speed Dynamics/1 -> Integrator/1
  Integrator/1 -> Vehicle Speed/1
  Acceleration Command/1 -> Vehicle Acc to Speed Dynamics/1

== system MOBATSim/Vehicle Model 6/Longitudinal Speed Control/Acceleration Command ==
  Driving Mode : Inport
  Speed Error : Inport  Port=2
  Actual Speed : Inport  Port=3
  Emergency Brake : Constant  Value=MinDeceleration
  Gear Logic : Stateflow chart  TreatAsAtomicUnit=on
  Multiport Switch3 : MultiPortSwitch  Inputs=4
  Saturation Dynamic : simulink/Discontinuities/Saturation Dynamic  OutMin=[]  OutMax=[]  OutDataTypeStr=Inherit: Same as second input  OutDataType=fixdt(1, 16)  OutScaling=2^-10  DoSatur=off
  Acceleration Command : Outport  VectorParamsAs1DForOutWhenUnconnected=off
  wires:
  Driving Mode/1 -> Multiport Switch3/1
  Speed Error/1 -> Saturation Dynamic/2
  Emergency Brake/1 -> Saturation Dynamic/3, Multiport Switch3/4
  Saturation Dynamic/1 -> Multiport Switch3/5, Multiport Switch3/2, Multiport Switch3/3
  Actual Speed/1 -> Gear Logic/1(speed)
  Multiport Switch3/1 -> Acceleration Command/1
  Gear Logic/1(maxAcc) -> Saturation Dynamic/1

== system MOBATSim/Vehicle Model 6/Longitudinal Speed Control/Distance to Stop Controller ==
  Speed Ref from Platoon : Inport
  Distance to Stop : Inport  Port=2
  Gain : Gain  Gain=0.02
  Multiport Switch2 : MultiPortSwitch  DataPortOrder=Zero-based contiguous  Inputs=2  zeroidx=on
  Relational Operator : RelationalOperator  Operator=<=  OutDataTypeStr=boolean  RndMeth=Simplest
  ref speed : Outport  VectorParamsAs1DForOutWhenUnconnected=off
  wires:
  Distance to Stop/1 -> Gain/1
  Speed Ref from Platoon/1 -> Relational Operator/1, Multiport Switch2/3
  Gain/1 -> Relational Operator/2, Multiport Switch2/2
  Multiport Switch2/1 -> ref speed/1
  Relational Operator/1 -> Multiport Switch2/1

== system MOBATSim/Vehicle Model 6/Longitudinal Speed Control/Platoon Controller ==
  Inter Vehicular Distance : Inport
  Lead Speed : Inport  Port=2
  Vehicle Speed : Inport  Port=3
  Compare To Constant : simulink/Logic and Bit Operations/Compare To Constant  relop=>  const=2  OutDataTypeStr=uint8
  Constant : Constant  Value=meters
  Gain : Gain  Gain=1.4
  Multiport Switch : MultiPortSwitch  DataPortOrder=Zero-based contiguous  Inputs=2  zeroidx=on
  PID Controller5 : simulink/Continuous/PID Controller  Controller=PID  Form=Parallel  TimeDomain=Continuous-time  UseExternalTs=off  SampleTime=-1  IntegratorMethod=Forward Euler  FilterMethod=Forward Euler  ControllerParametersSource=internal  P=2.0341199375219  I=0.0356576460366845  D=2.08363010404189  UseFilter=on  N=233.214579742572  TunerSelectOption=Transfer Function Based (PID Tuner App)  InitialConditionSource=internal  InitialConditionForIntegrator=0  InitialConditionForFilter=0  DifferentiatorICPrevScaledInput=0  ExternalReset=none  TrackingMode=off  Kt=1  LimitOutput=on  UpperSaturationLimit=100  LowerSaturationLimit=-100  LinearizeAsGain=on  AntiWindupMode=clamping  Kb=1  POutMin=[]  POutMax=[]  IOutMin=[]  IOutMax=[]  DOutMin=[]  DOutMax=[]  NOutMin=[]  NOutMax=[]  SumOutMin=[]  SumOutMax=[]  SaturationOutMin=[]  SaturationOutMax=[]  PParamMin=[]  PParamMax=[]  IParamMin=[]  IParamMax=[]  DParamMin=[]  DParamMax=[]  NParamMin=[]  NParamMax=[]  KbParamMin=[]  KbParamMax=[]  KtParamMin=[]  KtParamMax=[]  KbOutMin=[]  KbOutMax=[]  KtOutMin=[]  KtOutMax=[]  IntegratorOutMin=[]  IntegratorOutMax=[]  FilterOutMin=[]  FilterOutMax=[]  SumI1OutMin=[]  SumI1OutMax=[]  SumI2OutMin=[]  SumI2OutMax=[]  SumI3OutMin=[]  SumI3OutMax=[]  SumI4OutMin=[]  SumI4OutMax=[]  SumDOutMin=[]  SumDOutMax=[]  DifferentiatorOutMin=[]  DifferentiatorOutMax=[]  FilterDiffOutCoefMin=[]  FilterDiffOutCoefMax=[]  ReciprocalOutMin=[]  ReciprocalOutMax=[]  SumDenOutMin=[]  SumDenOutMax=[]  SumNumOutMin=[]  SumNumOutMax=[]  DivideOutMin=[]  DivideOutMax=[]  UdiffTsProdOutMin=[]  UdiffTsProdOutMax=[]  NTsProdOutMin=[]  NTsProdOutMax=[]  UintegralTsProdOutMin=[]  UintegralTsProdOutMax=[]  UngainTsProdOutMin=[]  UngainTsProdOutMax=[]  IntegratorContinuousStateAttributes=''  IntegratorStateMustResolveToSignalObject=off  IntegratorRTWStateStorageClass=Auto  FilterContinuousStateAttributes=''  FilterStateMustResolveToSignalObject=off  FilterRTWStateStorageClass=Auto  ParallelPVariant=InternalParameters  IdealPVariant=Disabled  IVariant=InternalParameters  DVariant=InternalParameters  IntegratorVariant=Continuous  SatVariant=Enabled  AWVariant=ContClampingParallel  PCopyVariant=Disabled  TRVariant=Disabled  FdbkBlocksVariant=Forward  IdealPFdbkVariant=Disabled  SatFdbkVariant=Disabled  DerivativeFilterVariant=ContFilter  NVariant=InternalParameters  NCopyVariant=Disabled  FilterICVariant=InternalICsFilter  IntegratorICVariant=InternalICs  ExternalResetVariant=Disabled  TRSumVariant=Passthrough  SumFdbkVariant=Disabled  SumVariant=Sum_PID  TsampFilterVariant=InternalTs  TsampNgainVariant=Passthrough  TsampIntegralVariant=Passthrough
  Sum : Sum  Inputs=|-+
  Sum1 : Sum  Inputs=|++
  Sum2 : Sum  Inputs=|+-
  Transfer Fcn : TransferFcn  Numerator=[0.05]  Denominator=[1 2]
  ref speed : Outport  VectorParamsAs1DForOutWhenUnconnected=off
  wires:
  Transfer Fcn/1 -> PID Controller5/1
  Vehicle Speed/1 -> Gain/1, Sum/1
  PID Controller5/1 -> Multiport Switch/2
  Sum/1 -> Compare To Constant/1
  Multiport Switch/1 -> ref speed/1
  Compare To Constant/1 -> Multiport Switch/1
  Lead Speed/1 -> Sum/2, Multiport Switch/3
  Constant/1 -> Sum1/1
  Sum1/1 -> Sum2/2
  Gain/1 -> Sum1/2
  Sum2/1 -> Transfer Fcn/1
  Inter Vehicular Distance/1 -> Sum2/1

== system MOBATSim/Vehicle Model 6/Longitudinal Speed Control/Reference speed according to the driving mode ==
  In1 : Inport
  In2 : Inport  Port=2
  In3 : Inport  Port=3
  In4 : Inport  Port=4
  Constant1 : Constant  Value=0
  Max Speed : Saturate  UpperLimit=maxSpeed  LowerLimit=-100
  Multiport Switch : MultiPortSwitch  Inputs=4
  Out1 : Outport
  wires:
  Constant1/1 -> Multiport Switch/4
  Multiport Switch/1 -> Max Speed/1
  In1/1 -> Multiport Switch/1
  In3/1 -> Multiport Switch/3
  In2/1 -> Multiport Switch/2
  Max Speed/1 -> Out1/1
  In4/1 -> Multiport Switch/5

== system MOBATSim/Vehicle Model 6/Longitudinal Speed Control/Vehicle Dynamic Model ==
  Acceleration Command : Inport
  Integrator : Integrator  LimitOutput=on  LowerSaturationLimit=0
  Vehicle Acc to Speed Dynamics : TransferFcn  Denominator=[0.5 1]
  Vehicle Speed : Outport
  wires:
  Vehicle Acc to Speed Dynamics/1 -> Integrator/1
  Integrator/1 -> Vehicle Speed/1
  Acceleration Command/1 -> Vehicle Acc to Speed Dynamics/1

== system MOBATSim/Vehicle Model 7/Longitudinal Speed Control/Acceleration Command ==
  Driving Mode : Inport
  Speed Error : Inport  Port=2
  Actual Speed : Inport  Port=3
  Emergency Brake : Constant  Value=MinDeceleration
  Gear Logic : Stateflow chart  TreatAsAtomicUnit=on
  Multiport Switch3 : MultiPortSwitch  Inputs=4
  Saturation Dynamic : simulink/Discontinuities/Saturation Dynamic  OutMin=[]  OutMax=[]  OutDataTypeStr=Inherit: Same as second input  OutDataType=fixdt(1, 16)  OutScaling=2^-10  DoSatur=off
  Acceleration Command : Outport  VectorParamsAs1DForOutWhenUnconnected=off
  wires:
  Driving Mode/1 -> Multiport Switch3/1
  Speed Error/1 -> Saturation Dynamic/2
  Emergency Brake/1 -> Saturation Dynamic/3, Multiport Switch3/4
  Saturation Dynamic/1 -> Multiport Switch3/5, Multiport Switch3/2, Multiport Switch3/3
  Actual Speed/1 -> Gear Logic/1(speed)
  Multiport Switch3/1 -> Acceleration Command/1
  Gear Logic/1(maxAcc) -> Saturation Dynamic/1

== system MOBATSim/Vehicle Model 7/Longitudinal Speed Control/Distance to Stop Controller ==
  Speed Ref from Platoon : Inport
  Distance to Stop : Inport  Port=2
  Gain : Gain  Gain=0.02
  Multiport Switch2 : MultiPortSwitch  DataPortOrder=Zero-based contiguous  Inputs=2  zeroidx=on
  Relational Operator : RelationalOperator  Operator=<=  OutDataTypeStr=boolean  RndMeth=Simplest
  ref speed : Outport  VectorParamsAs1DForOutWhenUnconnected=off
  wires:
  Distance to Stop/1 -> Gain/1
  Speed Ref from Platoon/1 -> Relational Operator/1, Multiport Switch2/3
  Gain/1 -> Relational Operator/2, Multiport Switch2/2
  Multiport Switch2/1 -> ref speed/1
  Relational Operator/1 -> Multiport Switch2/1
